simulink model "CiEngineController"  (R2019b)
settings: Solver=ode4  StartTime=0.0  StopTime=inf  FixedStep=.01  RelTol=1e-3  EnableMultiTasking=on
model workspace (MAT data in the model file):
  CatLightOffTime = 0
  Cps = 2
  EngRevLim = 6000
  EngStopStartEnable = 1
  EngStopTime = Simulink.Parameter
  EngStopTime.Value = 5
  EngStopTime.DataType = 'auto'
  EngStopTime.Dimensions = [1 1]
  NCyl = 4
  N_idle = 750
  Pstd = 101325
  Rair = 287.05
  Sinj = 6.45161290323
  Ts = Simulink.Parameter
  Ts.Value = 0.01
  Ts.DataType = 'auto'
  Ts.Dimensions = [1 1]
  Tstd = 293.15
  Vd = 0.0015
  afr_stoich = 14.6
  cp_exh = 1005
  f_egr_n_bpt = [0 500 750 1000 1250 1500 1750 2000 2250 2500 2750 3000 3250 3500 3750 4000]
  f_egr_stdflow = [0 0 0 0 0 0 0 0 0 0 0 0 ... (225 elements, 15x15)]
  f_egr_stdflow_egrap_bpt = [0 7.14285714286 14.2857142857 21.4285714286 28.5714285714 35.7142857143 42.8571428571 50 57.1428571429 64.2857142857 71.4285714286 78.5714285714 85.7142857143 92.8571428571 100]
  f_egr_stdflow_pr_bpt = [0.5 0.535714285714 0.571428571429 0.607142857143 0.642857142857 0.678571428571 0.714285714286 0.75 0.785714285714 0.821428571429 0.857142857143 0.892857142857 0.928571428571 0.964285714286 1]
  f_egr_tq_bpt = [10; 22.8571428571; 35.7142857143; 48.5714285714; 61.4285714286; 74.2857142857; 87.1428571429; 100; 112.857142857; 125.714285714; 138.571428571; 151.428571429; 164.285714286; 177.142857143; 190]
  f_egrcmd = [0 0 0 0 0 0 0 0 0 0 0 0 ... (240 elements, 15x16)]
  f_f_tot_n_bpt = [0 500 750 1000 1250 1500 1750 2000 2250 2500 2750 3000 3250 3500 3750 4000]
  f_f_tot_tq_bpt = [0; 12.6666666667; 25.3333333333; 38; 50.6666666667; 63.3333333333; 76; 88.6666666667; 101.333333333; 114; 126.666666667; 139.333333333; 152; 164.666666667; 177.333333333; 190]
  f_fcmd_tot = [0 6.79984066782 6.79984066782 6.79984066782 6.79984066782 6.79984066782 6.79984066782 6.79984066782 6.79984066782 6.79984066782 6.79984066782 6.79984066782 ... (256 elements, 16x16)]
  f_fric_temp_bpt = [275 277 279 281 283 285 287 289 291 293 295 297 299 301 303 305 307 309 311 313 315 317 319 321 323 325 327 329 331 333 335 337 339 341 343 345 347 349 351 353 355 357 359 361 363 365]
  f_fric_temp_mod = [3.986 2.616 2.132 1.946 1.839 1.747 1.672 1.608 1.551 1.499 1.462 1.415 1.363 1.314 1.275 1.248 1.223 1.195 1.173 1.15 1.134 1.113 1.097 1.082 1.065 1.051 1.039 1.025 1.01 1.001 0.9907 0.9802 0.9699 0.9595 0.9593 0.954 0.9415 0.9368 0.9285 0.923 0.9185 0.9093 0.9018 0.8989 0.8965 0.887]
  f_main_soi = [0 0 0 0 0 0 0 0 0 0 0 0 ... (240 elements, 15x16)]
  f_main_soi_f_bpt = [0; 3.57142857143; 7.14285714286; 10.7142857143; 14.2857142857; 17.8571428571; 21.4285714286; 25; 28.5714285714; 32.1428571429; 35.7142857143; 39.2857142857; 42.8571428571; 46.4285714286; 50]
  f_main_soi_n_bpt = [0 500 750 1000 1250 1500 1750 2000 2250 2500 2750 3000 3250 3500 3750 4000]
  f_nv = [0.954646224834 0.927678310575 0.901063682417 0.875710037198 0.852450535311 0.831986822876 0.814844392337 0.80134438932 0.791593989181 0.785495277781 0.782770492696 0.782999798686 ... (450 elements, 30x15)]
  f_nv_n_bpt = [1000 1285.71428571 1571.42857143 1857.14285714 2142.85714286 2428.57142857 2714.28571429 3000 3285.71428571 3571.42857143 3857.14285714 4142.85714286 4428.57142857 4714.28571429 5000]
  f_nv_prs_bpt = [95 100.344827586 105.689655172 111.034482759 116.379310345 121.724137931 127.068965517 132.413793103 137.75862069 143.103448276 148.448275862 153.793103448 159.137931034 164.482758621 169.827586207 175.172413793 180.517241379 185.862068966 191.206896552 196.551724138 201.896551724 207.24137931 212.586206897 217.931034483 223.275862069 228.620689655 233.965517241 239.310344828 244.655172414 250]
  f_rp_n_bpt = [0 500 750 1000 1250 1500 1750 2000 2250 2500 2750 3000 3250 3500 3750 4000]
  f_rp_tq_bpt = [10; 22.8571428571; 35.7142857143; 48.5714285714; 61.4285714286; 74.2857142857; 87.1428571429; 100; 112.857142857; 125.714285714; 138.571428571; 151.428571429; 164.285714286; 177.142857143; 190]
  f_rpcmd = [1 1 0.760752715621 0.597015667178 0.461549159226 0.363516478598 0.284701900288 0.203293429012 0.131191051 0.1 0.1 0.1 ... (240 elements, 15x16)]
  f_t_exh = [358.711368346 429.963145924 497.987869771 559.016510887 625.497016294 690.207854611 731.780908025 749.899407528 764.155922317 789.797182974 824.513264157 858.92580636 ... (240 elements, 16x15)]
  f_t_exh_f_bpt = [0 3.57 6.855 10.14 13.425 16.71 19.995 23.28 26.565 29.85 33.135 36.42 39.705 42.99 46.275 49.56]
  f_t_exh_n_bpt = [1000 1285.71428571 1571.42857143 1857.14285714 2142.85714286 2428.57142857 2714.28571429 3000 3285.71428571 3571.42857143 3857.14285714 4142.85714286 4428.57142857 4714.28571429 5000]
  f_tq_nf = [0 4.01032735147 17.4541547029 30.8399626872 43.6894710619 54.6724182266 65.9817429981 74.8844587697 82.0625281792 91.0474591726 100.604737295 107.761633858 ... (320 elements, 20x16)]
  f_tq_nf_f_bpt = [0 2.63157894737 5.26315789474 7.89473684211 10.5263157895 13.1578947368 15.7894736842 18.4210526316 21.0526315789 23.6842105263 26.3157894737 28.9473684211 31.5789473684 34.2105263158 36.8421052632 39.4736842105 42.1052631579 44.7368421053 47.3684210526 50]
  f_tq_nf_n_bpt = [0 1000 1285.71428571 1571.42857143 1857.14285714 2142.85714286 2428.57142857 2714.28571429 3000 3285.71428571 3571.42857143 3857.14285714 4142.85714286 4428.57142857 4714.28571429 5000]
  f_tqs_emap = [101325 101325 101325 101325 101325 101325 101325 101325 101325 101325 101325 101325 ... (240 elements, 15x16)]
  f_tqs_exht = [293.15 293.15 293.15 293.15 293.15 293.15 293.15 293.15 293.15 293.15 293.15 293.15 ... (240 elements, 15x16)]
  f_tqs_exht_fuelpress_eff = [1  1  1  1  1  1  1  1  1  1  1  1  1  1  1  1; 1  1  1  1  1  1  1  1  1  1  1  1  1  1  1  1; 1  1  1  1  1  1  1  1  1  1  1  1  1  1  1  1; 1  1  1  1  1  1  1  1  1  1  1  1  1  1  1  1; 1  1  1  1  1  1  1  1  1  1  1  1  1  1  1  1; 1  1  1  1  1  1  1  1  1  1  1  1  1  1  1  1; 1  1  1  1  1  1  1  1  1  1  1  1  1  1  1  1; 1  1  1  1  1  1  1  1  1  1  1  1  1  1  1  1; 1  1  1  1  1  1  1  1  1  1  1  1  1  1  1  1; 1  1  1  1  1  1  1  1  1  1  1  1  1  1  1  1; 1  1  1  1  1  1  1  1  1  1  1  1  1  1  1  1; 1  1  1  1  1  1  1  1  1  1  1  1  1  1  1  1; 1  1  1  1  1  1  1  1  1  1  1  1  1  1  1  1; 1  1  1  1  1  1  1  1  1  1  1  1  1  1  1  1; 1  1  1  1  1  1  1  1  1  1  1  1  1  1  1  1]
  f_tqs_exht_mainsoi_eff = [1 1 1 1 1 1 1 1 1 1 1 1 ... (240 elements, 15x16)]
  f_tqs_exht_map_eff = [1.11693337379 1.10383565741 1.07527138779 1.03804427558 1 0.975297725101 0.950398019177 0.924393698482 0.899021655666 0.876045599233 0.858573316119 0.844444824038 ... (225 elements, 15x15)]
  f_tqs_exht_mat_eff = [1 1 1 1 1 1 1 1 1 1 1 1 ... (240 elements, 15x16)]
  f_tqs_exht_o2pct_eff = [1 1 1 1 1 1 1 1 1 1 1 1 ... (240 elements, 15x16)]
  f_tqs_exht_post_inj_wall_htc = 0
  f_tqs_f_bpt = [0; 3.57142857143; 7.14285714286; 10.7142857143; 14.2857142857; 17.8571428571; 21.4285714286; 25; 28.5714285714; 32.1428571429; 35.7142857143; 39.2857142857; 42.8571428571; 46.4285714286; 50]
  f_tqs_f_burned_soi_limit = 500
  f_tqs_f_inj_type = 0
  f_tqs_f_post_sum_bpt = [0 3.57142857143 7.14285714286 10.7142857143 14.2857142857 17.8571428571 21.4285714286 25 28.5714285714 32.1428571429 35.7142857143 39.2857142857 42.8571428571 46.4285714286 50]
  f_tqs_fmep = [0 0 0 0 0 0 0 0 0 0 0 0 ... (240 elements, 15x16)]
  f_tqs_fric_temp_bpt = [273.15; 275.166037736; 277.182075472; 279.198113208; 281.214150943; 283.230188679; 285.246226415; 287.262264151; 289.278301887; 291.294339623; 293.310377358; 295.326415094; 297.34245283; 299.358490566; 301.374528302; 303.390566038; 305.406603774; 307.422641509; 309.438679245; 311.454716981; 313.470754717; 315.486792453; 317.502830189; 319.518867925; 321.53490566; 323.550943396; 325.566981132; 327.583018868; 329.599056604; 331.61509434; 333.631132075; 335.647169811; 337.663207547; 339.679245283; 341.695283019; 343.711320755; 345.727358491; 347.743396226; 349.759433962; 351.775471698; 353.791509434; 355.80754717; 357.823584906; 359.839622642; 361.855660377; 363.871698113; 365.887735849; 367.903773585; 369.919811321; 371.935849057; 373.951886792; 375.967924528; 377.983962264; 380]
  f_tqs_fric_temp_mod = [1 1 1 1 1 1 1 1 1 1 1 1 ... (864 elements, 54x16)]
  f_tqs_fuelpress = [100  100  100  100  100  100  100  100  100  100  100  100  100  100  100  100; 100  100  100  100  100  100  100  100  100  100  100  100  100  100  100  100; 100  100  100  100  100  100  100  100  100  100  100  100  100  100  100  100; 100  100  100  100  100  100  100  100  100  100  100  100  100  100  100  100; 100  100  100  100  100  100  100  100  100  100  100  100  100  100  100  100; 100  100  100  100  100  100  100  100  100  100  100  100  100  100  100  100; 100  100  100  100  100  100  100  100  100  100  100  100  100  100  100  100; 100  100  100  100  100  100  100  100  100  100  100  100  100  100  100  100; 100  100  100  100  100  100  100  100  100  100  100  100  100  100  100  100; 100  100  100  100  100  100  100  100  100  100  100  100  100  100  100  100; 100  100  100  100  100  100  100  100  100  100  100  100  100  100  100  100; 100  100  100  100  100  100  100  100  100  100  100  100  100  100  100  100; 100  100  100  100  100  100  100  100  100  100  100  100  100  100  100  100; 100  100  100  100  100  100  100  100  100  100  100  100  100  100  100  100; 100  100  100  100  100  100  100  100  100  100  100  100  100  100  100  100]
  f_tqs_fuelpress_delta_bpt = [-30; -25.7142857143; -21.4285714286; -17.1428571429; -12.8571428571; -8.57142857143; -4.28571428571; 0; 4.28571428571; 8.57142857143; 12.8571428571; 17.1428571429; 21.4285714286; 25.7142857143; 30]
  f_tqs_fuelpress_eff = [1  1  1  1  1  1  1  1  1  1  1  1  1  1  1  1; 1  1  1  1  1  1  1  1  1  1  1  1  1  1  1  1; 1  1  1  1  1  1  1  1  1  1  1  1  1  1  1  1; 1  1  1  1  1  1  1  1  1  1  1  1  1  1  1  1; 1  1  1  1  1  1  1  1  1  1  1  1  1  1  1  1; 1  1  1  1  1  1  1  1  1  1  1  1  1  1  1  1; 1  1  1  1  1  1  1  1  1  1  1  1  1  1  1  1; 1  1  1  1  1  1  1  1  1  1  1  1  1  1  1  1; 1  1  1  1  1  1  1  1  1  1  1  1  1  1  1  1; 1  1  1  1  1  1  1  1  1  1  1  1  1  1  1  1; 1  1  1  1  1  1  1  1  1  1  1  1  1  1  1  1; 1  1  1  1  1  1  1  1  1  1  1  1  1  1  1  1; 1  1  1  1  1  1  1  1  1  1  1  1  1  1  1  1; 1  1  1  1  1  1  1  1  1  1  1  1  1  1  1  1; 1  1  1  1  1  1  1  1  1  1  1  1  1  1  1  1]
  f_tqs_imep_post_corr = [0  0  0  0  0  0  0  0  0  0  0  0  0  0  0; 0  0  0  0  0  0  0  0  0  0  0  0  0  0  0; 0  0  0  0  0  0  0  0  0  0  0  0  0  0  0; 0  0  0  0  0  0  0  0  0  0  0  0  0  0  0; 0  0  0  0  0  0  0  0  0  0  0  0  0  0  0; 0  0  0  0  0  0  0  0  0  0  0  0  0  0  0; 0  0  0  0  0  0  0  0  0  0  0  0  0  0  0; 0  0  0  0  0  0  0  0  0  0  0  0  0  0  0; 0  0  0  0  0  0  0  0  0  0  0  0  0  0  0; 0  0  0  0  0  0  0  0  0  0  0  0  0  0  0; 0  0  0  0  0  0  0  0  0  0  0  0  0  0  0; 0  0  0  0  0  0  0  0  0  0  0  0  0  0  0; 0  0  0  0  0  0  0  0  0  0  0  0  0  0  0; 0  0  0  0  0  0  0  0  0  0  0  0  0  0  0; 0  0  0  0  0  0  0  0  0  0  0  0  0  0  0]
  f_tqs_imepg = [0 158686.534722 343074.265588 507983.203346 653190.552872 792520.266872 898623.174707 1024926.34814 1192408.65419 1362289.29874 1538616.81914 1722468.1753 ... (240 elements, 15x16)]
  f_tqs_lambda_bpt = [1.5 1.67857142857 1.85714285714 2.03571428571 2.21428571429 2.39285714286 2.57142857143 2.75 2.92857142857 3.10714285714 3.28571428571 3.46428571429 3.64285714286 3.82142857143 4]
  f_tqs_mainsoi = [-5.65203706782 -5.56485950617 -5.32737749535 -4.90693102774 -4.39157989496 -2.6685350622 -1.13269707429 -0.442811837066 0.0846384555918 0.793458776955 1.62426195607 2.45698560821 ... (240 elements, 15x16)]
  f_tqs_mainsoi_delta_bpt = [-15; -12.8571428571; -10.7142857143; -8.57142857143; -6.42857142857; -4.28571428571; -2.14285714286; 0; 2.14285714286; 4.28571428571; 6.42857142857; 8.57142857143; 10.7142857143; 12.8571428571; 15]
  f_tqs_mainsoi_eff = [1 1 1 1 1 1 1 1 1 1 1 1 ... (240 elements, 15x16)]
  f_tqs_map = [101325 101325 101325 101325 101325 101325 101325 101325 101325 101325 101325 101325 ... (240 elements, 15x16)]
  f_tqs_map_eff = [0.876486797315 0.914614445767 0.94792295911 0.975703338034 1 1.02743787204 1.05216674291 1.07395048632 1.09371107566 1.11066007626 1.12521245816 1.14202789912 ... (225 elements, 15x15)]
  f_tqs_map_ratio_bpt = [0.8; 0.85; 0.9; 0.95; 1; 1.05; 1.1; 1.15; 1.2; 1.25; 1.3; 1.35; 1.4; 1.45; 1.5]
  f_tqs_mat = [293.15 293.15 293.15 293.15 293.15 293.15 293.15 293.15 293.15 293.15 293.15 293.15 ... (240 elements, 15x16)]
  f_tqs_mat_delta_bpt = [-55; -50; -45; -40; -35; -30; -25; -20; -15; -10; -5; 0; 5; 10; 15]
  f_tqs_mat_eff = [1 1 1 1 1 1 1 1 1 1 1 1 ... (240 elements, 15x16)]
  f_tqs_n_bpt = [0 500 750 1000 1250 1500 1750 2000 2250 2500 2750 3000 3250 3500 3750 4000]
  f_tqs_o2pct = [18.6138636402 19.5619833676 20.7378306586 22.1536730517 23.4120452691 23.8418651452 23.8693762547 23.8866954757 24.0193105899 24.2672589018 24.5893674985 24.9537951111 ... (240 elements, 15x16)]
  f_tqs_o2pct_delta_bpt = [-2; -1.33333333333; -0.666666666667; 0; 0.666666666667; 1.33333333333; 2; 2.66666666667; 3.33333333333; 4; 4.66666666667; 5.33333333333; 6; 6.66666666667; 7.33333333333]
  f_tqs_o2pct_eff = [1 1 1 1 1 1 1 1 1 1 1 1 ... (240 elements, 15x16)]
  f_tqs_pmep = [0 0 0 0 0 0 0 0 0 0 0 0 ... (240 elements, 15x16)]
  f_tqs_soi_post_cent_bpt = [150 160.714285714 171.428571429 182.142857143 192.857142857 203.571428571 214.285714286 225 235.714285714 246.428571429 257.142857143 267.857142857 278.571428571 289.285714286 300]
  f_turbo_pr = [1 1 1.00366494858 1.00841236661 1.01669032671 1.02766916175 1.04245504306 1.0631733336 1.08916626118 1.1150966519 1.13221323152 1.13265585874 ... (225 elements, 15x15)]
  f_turbo_pr_corrspd_bpt = [30 556.428571429 1082.85714286 1609.28571429 2135.71428571 2662.14285714 3188.57142857 3715 4241.42857143 4767.85714286 5294.28571429 5820.71428571 6347.14285714 6873.57142857 7400]
  f_turbo_pr_stdflow_bpt = [3 7.07142857143 11.1428571429 15.2142857143 19.2857142857 23.3571428571 27.4285714286 31.5 35.5714285714 39.6428571429 43.7142857143 47.7857142857 51.8571428571 55.9285714286 60]
  f_turbo_pr_vgtposcorr = [1.02855954111; 1.02335294047; 1.0182251931; 1.01353160145; 1.00975100162; 1.00744452152; 1.00702711526; 1.00854725935; 1.01183484525; 1.0163858771; 1.02148385659; 1.0270522279; 1.03306395358; 1.03926964489; 1.04548847114]
  f_turbo_pr_vgtposcorr_bpt = [0.1; 0.164285714286; 0.228571428571; 0.292857142857; 0.357142857143; 0.421428571429; 0.485714285714; 0.55; 0.614285714286; 0.678571428571; 0.742857142857; 0.807142857143; 0.871428571429; 0.935714285714; 1]
  fuel_lhv = 42000000
libraries: simulink x3, autolibengctrlr x1
(part 1 of 2)
settings Model: ModifiedByFormat=The MathWorks, Inc.  OrderedModelArguments=off  Creator=The MathWorks, Inc.  LastModifiedBy=The MathWorks, Inc.
settings DataIOCC: DSMLogging=off  ReturnWorkspaceOutputs=off
settings DebuggingCC: PregeneratedLibrarySubsystemCodeDiagnostic=none  ArithmeticOperatorsInVariantConditions=warning
settings SFSimCC: SimUseLocalCustomCode=off  CustomCodeUndefinedFunction=UseInterfaceOnly
settings RTWCC: RTWUseLocalCustomCode=off
settings CodeAppCC: StateflowObjectComments=on
settings GRTTargetCC: TargetLangStandard=C89/C90 (ANSI)
settings ConfigComp: CovMetricSettings=dsw  CovHtmlReporting=on  CovSaveCumulativeToWorkspaceVar=on  CovSaveSingleToWorkspaceVar=on  CovShowResultsExplorer=off  CovExternalEMLEnable=off

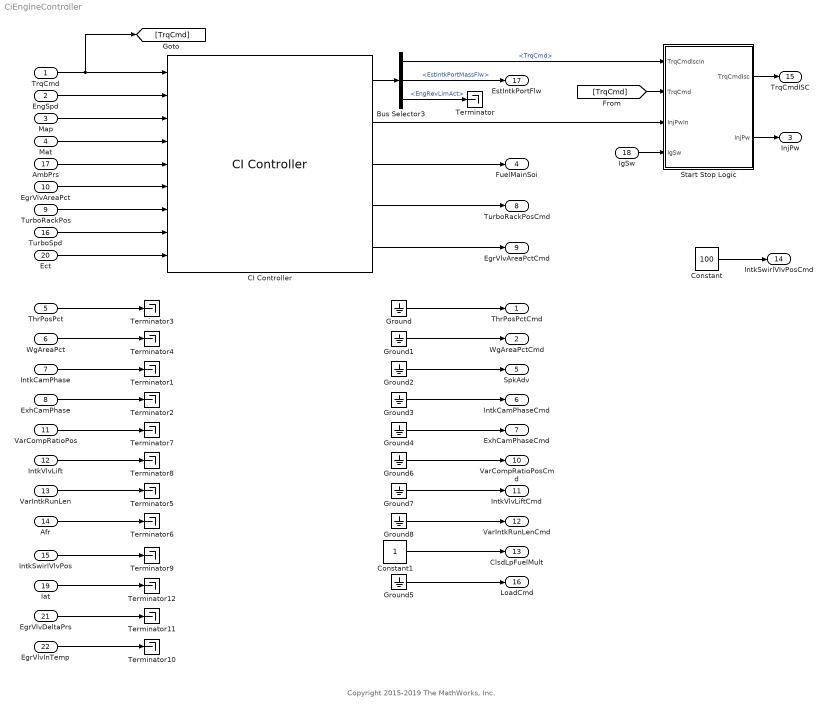
== system CiEngineController ==
  note: Copyright 2015-2019 The MathWorks, Inc.
  TrqCmd : Inport
  EngSpd : Inport  Port=2
  Map : Inport  Port=3
  Mat : Inport  Port=4
  ThrPosPct : Inport  Port=5  Unit=%
  WgAreaPct : Inport  Port=6  Unit=%
  IntkCamPhase : Inport  Port=7  Unit=deg
  ExhCamPhase : Inport  Port=8  Unit=deg
  TurboRackPos : Inport  Port=9
  EgrVlvAreaPct : Inport  Port=10
  VarCompRatioPos : Inport  Port=11
  IntkVlvLift : Inport  Port=12
  VarIntkRunLen : Inport  Port=13
  Afr : Inport  Port=14  Unit=1
  IntkSwirlVlvPos : Inport  Port=15
  TurboSpd : Inport  Port=16
  AmbPrs : Inport  Port=17
  IgSw : Inport  Port=18
  Iat : Inport  Port=19  Unit=K
  Ect : Inport  Port=20  Unit=K
  EgrVlvDeltaPrs : Inport  Port=21  Unit=Pa
  EgrVlvInTemp : Inport  Port=22  Unit=K
  Bus Selector3 : BusSelector  OutputSignals=TrqCmd,EstIntkPortMassFlw,EngRevLimAct
  CI Controller : autolibengctrlr/CI Controller  TrqEstOptionPopup=Torque Structure  f_egrcmd=f_egrcmd  f_egr_tq_bpt=f_egr_tq_bpt  f_egr_n_bpt=f_egr_n_bpt  f_rpcmd=f_rpcmd  f_rp_tq_bpt=f_rp_tq_bpt  f_rp_n_bpt=f_rp_n_bpt  Sinj=Sinj  afr_stoich=afr_stoich  fuel_lhv=fuel_lhv  f_fcmd_tot=f_fcmd_tot  f_main_soi=f_main_soi  f_main_soi_f_bpt=f_main_soi_f_bpt  f_main_soi_n_bpt=f_main_soi_n_bpt  f_f_tot_tq_bpt=f_f_tot_tq_bpt  f_f_tot_n_bpt=f_f_tot_n_bpt  N_idle=N_idle  Trq_idlecmd_enable=1  Trq_idlecmd_max=50  Kp_idle=0.1  Ki_idle=0.05  EngRevLim=EngRevLim  NCyl=NCyl  Cps=Cps  Vd=Vd  Rair=Rair  Pstd=Pstd  Tstd=Tstd  f_nv=f_nv  f_nv_prs_bpt=f_nv_prs_bpt  f_nv_n_bpt=f_nv_n_bpt  f_egr_stdflow=f_egr_stdflow  f_egr_stdflow_pr_bpt=f_egr_stdflow_pr_bpt  f_egr_stdflow_egrap_bpt=f_egr_stdflow_egrap_bpt  f_turbo_pr=f_turbo_pr  f_turbo_pr_stdflow_bpt=f_turbo_pr_stdflow_bpt  f_turbo_pr_corrspd_bpt=f_turbo_pr_corrspd_bpt  f_turbo_pr_vgtposcorr=f_turbo_pr_vgtposcorr  f_turbo_pr_vgtposcorr_bpt=f_turbo_pr_vgtposcorr_bpt  f_tq_nf=f_tq_nf  f_tq_nf_f_bpt=f_tq_nf_f_bpt  f_tq_nf_n_bpt=f_tq_nf_n_bpt  f_tqs_f_bpt=f_tqs_f_bpt  f_tqs_n_bpt=f_tqs_n_bpt  f_tqs_mainsoi=f_tqs_mainsoi  f_tqs_map=f_tqs_map  f_tqs_emap=f_tqs_emap  f_tqs_mat=f_tqs_mat  f_tqs_o2pct=f_tqs_o2pct  f_tqs_fuelpress=f_tqs_fuelpress  f_tqs_imepg=f_tqs_imepg  f_tqs_fmep=f_tqs_fmep  f_tqs_pmep=f_tqs_pmep  f_tqs_fric_temp_mod=f_tqs_fric_temp_mod  f_tqs_fric_temp_bpt=f_tqs_fric_temp_bpt  f_tqs_mainsoi_eff=f_tqs_mainsoi_eff  f_tqs_mainsoi_delta_bpt=f_tqs_mainsoi_delta_bpt  f_tqs_map_eff=f_tqs_map_eff  f_tqs_map_ratio_bpt=f_tqs_map_ratio_bpt  f_tqs_lambda_bpt=f_tqs_lambda_bpt  f_tqs_mat_eff=f_tqs_mat_eff  f_tqs_mat_delta_bpt=f_tqs_mat_delta_bpt  f_tqs_o2pct_eff=f_tqs_o2pct_eff  f_tqs_o2pct_delta_bpt=f_tqs_o2pct_delta_bpt  f_tqs_fuelpress_eff=f_tqs_fuelpress_eff  f_tqs_fuelpress_delta_bpt=f_tqs_fuelpress_delta_bpt  f_tqs_f_inj_type=f_tqs_f_inj_type  f_tqs_imep_post_corr=f_tqs_imep_post_corr  f_tqs_f_post_sum_bpt=f_tqs_f_post_sum_bpt  f_tqs_soi_post_cent_bpt=f_tqs_soi_post_cent_bpt  f_tqs_f_burned_soi_limit=f_tqs_f_burned_soi_limit  cp_exh=cp_exh  f_t_exh=f_t_exh  f_t_exh_f_bpt=f_t_exh_f_bpt  f_t_exh_n_bpt=f_t_exh_n_bpt  f_tqs_exht=f_tqs_exht  f_tqs_exht_mainsoi_eff=f_tqs_exht_mainsoi_eff  f_tqs_exht_map_eff=f_tqs_exht_map_eff  f_tqs_exht_mat_eff=f_tqs_exht_mat_eff  f_tqs_exht_o2pct_eff=f_tqs_exht_o2pct_eff  f_tqs_exht_fuelpress_eff=f_tqs_exht_fuelpress_eff  f_tqs_exht_post_inj_wall_htc=f_tqs_exht_post_inj_wall_htc
      settings: SourceProductName=Powertrain Blockset  SourceProductBaseCode=PW
  Constant : Constant  Value=100
  Constant1 : Constant
  Ground{,1..8} (9 alike) : Ground
  Start Stop Logic : Subsystem  TreatAsAtomicUnit=on
  Terminator{,1..12} (13 alike) : Terminator
  ThrPosPctCmd : Outport  Unit=%  VectorParamsAs1DForOutWhenUnconnected=off
  WgAreaPctCmd : Outport  Port=2  Unit=%  VectorParamsAs1DForOutWhenUnconnected=off
  InjPw : Outport  Port=3  Unit=ms  VectorParamsAs1DForOutWhenUnconnected=off
  FuelMainSoi : Outport  Port=4  VectorParamsAs1DForOutWhenUnconnected=off
  SpkAdv : Outport  Port=5  Unit=deg  VectorParamsAs1DForOutWhenUnconnected=off
  IntkCamPhaseCmd : Outport  Port=6  Unit=deg  VectorParamsAs1DForOutWhenUnconnected=off
  ExhCamPhaseCmd : Outport  Port=7  Unit=deg  VectorParamsAs1DForOutWhenUnconnected=off
  TurboRackPosCmd : Outport  Port=8  VectorParamsAs1DForOutWhenUnconnected=off
  EgrVlvAreaPctCmd : Outport  Port=9  VectorParamsAs1DForOutWhenUnconnected=off
  VarCompRatioPosCmd : Outport  Port=10  VectorParamsAs1DForOutWhenUnconnected=off
  IntkVlvLiftCmd : Outport  Port=11  VectorParamsAs1DForOutWhenUnconnected=off
  VarIntkRunLenCmd : Outport  Port=12  VectorParamsAs1DForOutWhenUnconnected=off
  ClsdLpFuelMult : Outport  Port=13  Unit=1  VectorParamsAs1DForOutWhenUnconnected=off
  IntkSwirlVlvPosCmd : Outport  Port=14  VectorParamsAs1DForOutWhenUnconnected=off
  TrqCmdISC : Outport  Port=15  Unit=N*m  VectorParamsAs1DForOutWhenUnconnected=off
  LoadCmd : Outport  Port=16  Unit=1  VectorParamsAs1DForOutWhenUnconnected=off
  EstIntkPortFlw : Outport  Port=17  Unit=kg/s  VectorParamsAs1DForOutWhenUnconnected=off
  wires:
  AmbPrs/1 -> CI Controller/5
  Map/1 -> CI Controller/3
  Mat/1 -> CI Controller/4
  IntkCamPhase/1 -> Terminator1/1
  ExhCamPhase/1 -> Terminator2/1
  CI Controller/1 -> Bus Selector3/1
  EngSpd/1 -> CI Controller/2
  Ground/1 -> ThrPosPctCmd/1
  TrqCmd/1 -> [TrqCmd], CI Controller/1
  Bus Selector3/1 -> Start Stop Logic/1(TrqCmdIscIn)  "<TrqCmd>"
  CI Controller/4 -> TurboRackPosCmd/1
  CI Controller/5 -> EgrVlvAreaPctCmd/1
  Ground1/1 -> WgAreaPctCmd/1
  Ground2/1 -> SpkAdv/1
  Ground3/1 -> IntkCamPhaseCmd/1
  Ground4/1 -> ExhCamPhaseCmd/1
  Bus Selector3/2 -> EstIntkPortFlw/1  "<EstIntkPortMassFlw>"
  Ground5/1 -> LoadCmd/1
  CI Controller/3 -> FuelMainSoi/1
  EgrVlvAreaPct/1 -> CI Controller/6
  TurboRackPos/1 -> CI Controller/7
  TurboSpd/1 -> CI Controller/8
  CI Controller/2 -> Start Stop Logic/3(InjPwIn)
  Start Stop Logic/2(InjPw) -> InjPw/1
  [TrqCmd] -> Start Stop Logic/2(TrqCmd)
  Start Stop Logic/1(TrqCmdIsc) -> TrqCmdISC/1
  Ground6/1 -> VarCompRatioPosCmd/1
  Ground7/1 -> IntkVlvLiftCmd/1
  Ground8/1 -> VarIntkRunLenCmd/1
  Constant1/1 -> ClsdLpFuelMult/1
  Constant/1 -> IntkSwirlVlvPosCmd/1
  WgAreaPct/1 -> Terminator4/1
  ThrPosPct/1 -> Terminator3/1
  VarCompRatioPos/1 -> Terminator7/1
  IntkVlvLift/1 -> Terminator8/1
  Afr/1 -> Terminator6/1
  VarIntkRunLen/1 -> Terminator5/1
  IntkSwirlVlvPos/1 -> Terminator9/1
  IgSw/1 -> Start Stop Logic/4(IgSw)
  Ect/1 -> CI Controller/9
  Iat/1 -> Terminator12/1
  EgrVlvInTemp/1 -> Terminator10/1
  EgrVlvDeltaPrs/1 -> Terminator11/1
  Bus Selector3/3 -> Terminator/1  "<EngRevLimAct>"
